simulink model "simulink1"  (R2016a)
settings: Solver=VariableStepAuto  StartTime=0.0  StopTime=10.0  RelTol=1e-3
settings Model: Creator=user  LastModifiedBy=user

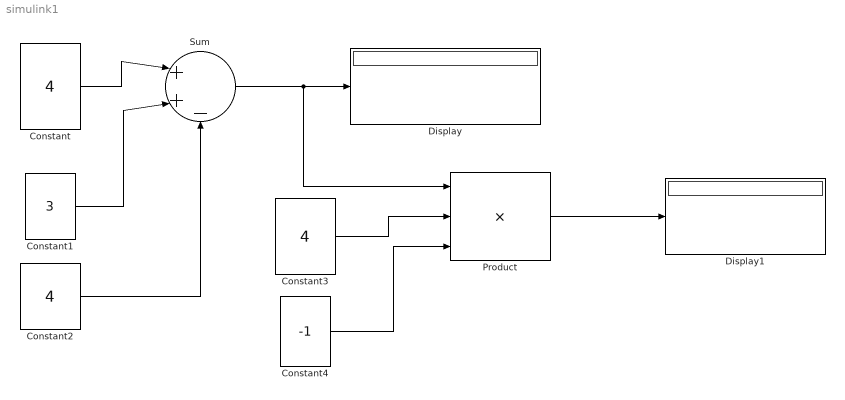
== system simulink1 ==
  Constant : Constant  Value=4
  Constant1 : Constant  Value=3
  Constant2 : Constant  Value=4
  Constant3 : Constant  Value=4
  Constant4 : Constant  Value=-1
  Display : Display
  Display1 : Display
  Product : Product  Inputs=3
  Sum : Sum  Inputs=|++-
  wires:
  Constant/1 -> Sum/1
  Constant1/1 -> Sum/2
  Constant2/1 -> Sum/3
  Sum/1 -> Product/1, Display/1
  Constant3/1 -> Product/2
  Constant4/1 -> Product/3
  Product/1 -> Display1/1
